simulink model "powerwindow_tl_v04"  (R2021a)
settings: Solver=ode1  StartTime=0.0  StopTime=20.0  FixedStep=0.01  RelTol=1e-3
PreLoadFcn:
  | if exist('tl_preloadfcn','file'), tl_preloadfcn(gcs,'22.1.0.27'); end
PostLoadFcn:
  | if exist('tl_postloadfcn','file'), tl_postloadfcn(gcs,'22.1.0.27'); end
InitFcn:
  | if exist('tlds_init','file'), tlds_init(gcs); end
StartFcn:
  | if exist('tlds_start','file'), tlds_start(gcs); end
StopFcn:
  | if exist('tlds_stop','file'), tlds_stop(gcs); end
undefined symbols (not defined in the file): auto_down_time, auto_up_time, emergency_down_time, position_endstop_top
libraries: tllib x7
(part 1 of 2)
PreSaveFcn:
  | if exist('tl_presavefcn','file'), tl_presavefcn(gcs); end
CloseFcn:
  | if exist('tl_closefcn','file'), tl_closefcn(gcs); end
settings Model: TL_MAIN_DATA={'codeopt',{'cleancode',1},'date',738946.6185320717,'advcodeopt',{'ExtendedBlockComments';'true'}}  DS_PROJECTFILE=powerwindow_tl_v01.dd  TLVersion=22.1.0.27  TL_GLOBAL_LOGGING_MODE=4  Creator=Wolfgang Meincke  LastModifiedBy=yatishc
settings SolverCC: AlgebraicLoopSolver=TrustRegion
settings DataIOCC: LimitDataPoints=on  SaveFormat=Array  ReturnWorkspaceOutputs=off
settings OptimizationCC: BlockReduction=off  BooleanDataType=off  ConditionallyExecuteInputs=off  OptimizeBlockIOStorage=off  BufferReuse=off  GlobalBufferReuse=off  ExpressionFolding=off  ExpressionDepthLimit=2147483647  LocalBlockOutputs=off  LifeSpan=inf  OptimizeDataStoreBuffers=off  BusAssignmentInplaceUpdate=off
settings DebuggingCC: SaveWithParameterizedLinksMsg=none  UnderspecifiedInitializationDetection=Classic  MergeDetectMultiDrivingBlocksExec=none  MultiTaskDSMMsg=warning  MultiTaskCondExecSysMsg=none  FcnCallInpInsideContextMsg=warning  UnconnectedInputMsg=none  UnconnectedOutputMsg=none  BusObjectLabelMismatch=error  StateNameClashWarn=warning  StrictBusMsg=ErrorOnBusTreatedAsVector  NonBusSignalsTreatedAsBus=error  SFUnexpectedBacktrackingDiag=warning  SFNoUnconditionalDefaultTransitionDiag=warning  SFMachineParentedDataDiag=warning  ArithmeticOperatorsInVariantConditions=warning
settings HardwareCC: ProdBitPerPointer=32  ProdBitPerSizeT=32  ProdBitPerPtrDiffT=32  ProdLargestAtomicFloat=None  ProdIntDivRoundTo=Undefined  ProdEndianess=Unspecified  ProdWordSize=32  ProdHWDeviceType=32-bit Generic
settings ModelReferenceCC: PropagateSignalLabelsOutOfModel=off
settings SFSimCC: SimUseLocalCustomCode=off  SimParseCustomCode=off  CustomCodeUndefinedFunction=UseInterfaceOnly
settings RTWCC: RTWUseLocalCustomCode=off
settings CodeAppCC: StateflowObjectComments=on
settings GRTTargetCC: TargetLangStandard=C89/C90 (ANSI)  CombineOutputUpdateFcns=off  GRTInterface=on
settings ConfigComp: CovMetricSettings=dw  CovSaveCumulativeToWorkspaceVar=on  CovSaveSingleToWorkspaceVar=on  CovExternalEMLEnable=off  CovSFcnEnable=off

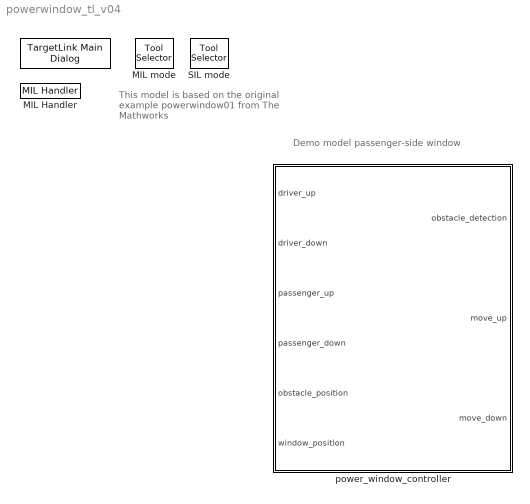
== system powerwindow_tl_v04 ==
  note: Demo model passenger-side window
  note: This model is based on the
      | original example powerwindow01
      | from The Mathworks
  " " : tllib/TargetLink Main Dialog  data=[]
      settings: SourceProductName=dSPACE TargetLink common blockset
  MIL Handler : tllib/MIL Handler  data={'date',730486}
      settings: SourceProductName=dSPACE TargetLink common blockset
  MIL mode : tllib/Tool Selector  Description=MIL\nmode  data={'date',730486}
      settings: SourceProductName=dSPACE TargetLink common blockset
  SIL mode : tllib/Tool Selector  Description=SIL\nmode  data={'date',730486}
      settings: SourceProductName=dSPACE TargetLink common blockset
  power_window_controller : Subsystem  Tag=TargetLink Simulation Frame  mask(TL_SimFrame){}
      settings: CopyFcn=if exist('tl_copyfcn','file'), tl_copyfcn(gcbh); end  NameChangeFcn=if exist('tl_framenamechangefcn','file'), tl_framenamechangefcn(gcbh); end
      settings: OpenFcn=|
      | if exist('open_tlsubsystem','file')
      |    open_tlsubsystem(gcbh);
      | else
      |    tlsubsystem = ...
      |       find_system(gcb, ...
      |       'LookUnderMasks','on', ...
      |       'FollowLinks','on', ...
      |       'Tag','MIL Subsystem');
      |    open_system(tlsubsystem);
      | end
      mask Display: disp('TargetLink\nModel-\nin-the-loop\nmode')

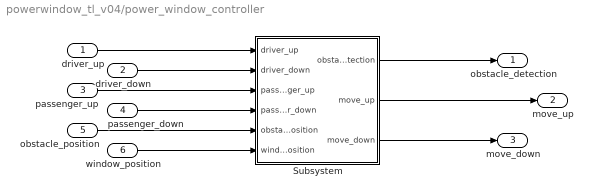
== system powerwindow_tl_v04/power_window_controller ==
  driver_up : Inport
  driver_down : Inport  Port=2
  passenger_up : Inport  Port=3
  passenger_down : Inport  Port=4
  obstacle_position : Inport  Port=5
  window_position : Inport  Port=6
  Subsystem : Subsystem  Tag=struct('sfcnName','power_window_controller_sf','subFunction','','srcSubsystem','')  mask(TL_Enable){}
      settings: OpenFcn=warndlg(get_param(gcb,'MaskHelp'),'Serious Warning');
      mask Help: This subsystem keeps the TargetLink subsystem (subsystem with TargetLink blocks for production code generation), and is needed for the TargetLink simulation frame to work properly. DO NOT DELETE OR MODIFY IT!
  obstacle_detection : Outport
  move_up : Outport  Port=2
  move_down : Outport  Port=3
  wires:
  driver_up/1 -> Subsystem/1(driver_up)
  driver_down/1 -> Subsystem/2(driver_down)
  passenger_up/1 -> Subsystem/3(passenger_up)
  passenger_down/1 -> Subsystem/4(passenger_down)
  obstacle_position/1 -> Subsystem/5(obstacle_position)
  window_position/1 -> Subsystem/6(window_position)
  Subsystem/1(obstacle_detection) -> obstacle_detection/1
  Subsystem/2(move_up) -> move_up/1
  Subsystem/3(move_down) -> move_down/1

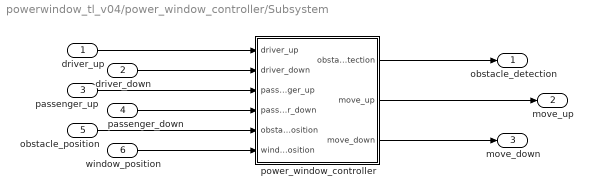
== system powerwindow_tl_v04/power_window_controller/Subsystem ==
  driver_up : Inport
  driver_down : Inport  Port=2
  passenger_up : Inport  Port=3
  passenger_down : Inport  Port=4
  obstacle_position : Inport  Port=5
  window_position : Inport  Port=6
  power_window_controller : Subsystem  Tag=MIL Subsystem  Description=a  RequirementInfo={} %GIDa_af814551_25fe_45fb_8d1f_eceee28b4185  LoadFcn=|
      | if exist('TargetLink.SimFrameHandler.TLSubsystem','class')
      |     TargetLink.SimFrameHandler.TLSubsystem.CreateWatchDog(gcbh);
      | end
      settings: CopyFcn=if exist('tl_copyfcn','file'), tl_copyfcn(gcbh); end  NameChangeFcn=if exist('tl_namechangefcn','file'), tl_namechangefcn(gcbh); end  DestroyFcn=if exist('update_tl_main_dlg','file'), update_tl_main_dlg('TL_subs_display'); end
      mask Display: disp('TargetLink Subsystem')
  obstacle_detection : Outport
  move_up : Outport  Port=2
  move_down : Outport  Port=3
  wires:
  driver_up/1 -> power_window_controller/1(driver_up)
  driver_down/1 -> power_window_controller/2(driver_down)
  passenger_up/1 -> power_window_controller/3(passenger_up)
  passenger_down/1 -> power_window_controller/4(passenger_down)
  obstacle_position/1 -> power_window_controller/5(obstacle_position)
  window_position/1 -> power_window_controller/6(window_position)
  power_window_controller/1(obstacle_detection) -> obstacle_detection/1
  power_window_controller/2(move_up) -> move_up/1
  power_window_controller/3(move_down) -> move_down/1

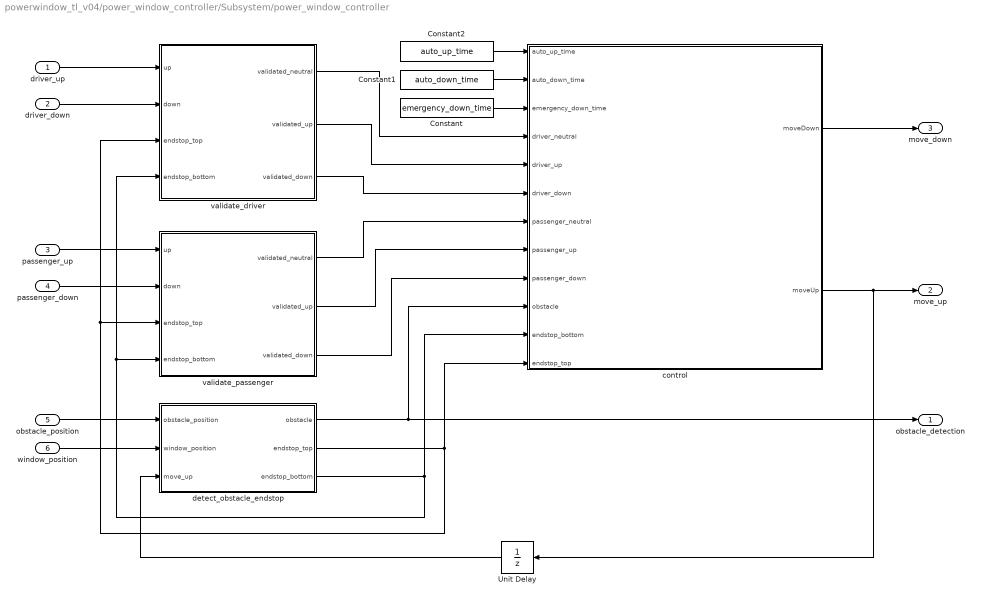
== system powerwindow_tl_v04/power_window_controller/Subsystem/power_window_controller ==
  driver_up : Inport  RequirementInfo={} %GIDa_659446e1_8e6d_43f9_b2fb_39d8267d7cb4  PortDimensions=1  mask(TL_Inport){data={'output',{'variable','Interface_Variables/driver_up'},'date',737859.75098331016}}
      settings: CopyFcn=if exist('copy_tlblock','file')==2,copy_tlblock(gcbh);end  DeleteFcn=if exist('delete_tlblock','file')==2,delete_tlblock(gcbh);end  NameChangeFcn=if exist('rename_tlblock','file')==2,rename_tlblock(gcbh);end  OpenFcn=if exist('tl_open_blockdlg','file')==2,tl_open_blockdlg(gcbh);else,open_system(gcbh,'parameter');end
      mask Help: eval(['if exist(''tl_online_help'',''file'') == 2, tl_online_help(''Topic'',''TL_Inport''),else, web([''jar:file:///'',matlabroot,''/help/toolbox/simulink/help.jar!/slref/' lower(get_param(gcbh,'Blocktype')) '.html''], ''-helpbrowser''),end'])
      mask Display:
      | [x,y] = tlDrawBrandOnBlockIcon(gcbh);
      | plot(x,y);
  driver_down : Inport  RequirementInfo={} %GIDa_1ab93b35_c370_40d7_8cfb_ac38c79443a8  Port=2  PortDimensions=1  mask(TL_Inport){data={'output',{'variable','Interface_Variables/driver_down'},'date',737859.75098344905}}
      settings: CopyFcn=if exist('copy_tlblock','file')==2,copy_tlblock(gcbh);end  DeleteFcn=if exist('delete_tlblock','file')==2,delete_tlblock(gcbh);end  NameChangeFcn=if exist('rename_tlblock','file')==2,rename_tlblock(gcbh);end  OpenFcn=if exist('tl_open_blockdlg','file')==2,tl_open_blockdlg(gcbh);else,open_system(gcbh,'parameter');end
      mask Help: eval(['if exist(''tl_online_help'',''file'') == 2, tl_online_help(''Topic'',''TL_Inport''),else, web([''jar:file:///'',matlabroot,''/help/toolbox/simulink/help.jar!/slref/' lower(get_param(gcbh,'Blocktype')) '.html''], ''-helpbrowser''),end'])
      mask Display:
      | [x,y] = tlDrawBrandOnBlockIcon(gcbh);
      | plot(x,y);
  passenger_up : Inport  RequirementInfo={} %GIDa_d69b69e4_dcf8_4d19_8e10_903162015345  Port=3  PortDimensions=1  mask(TL_Inport){data={'output',{'variable','Interface_Variables/passenger_up'},'date',737859.75098356477}}
      settings: CopyFcn=if exist('copy_tlblock','file')==2,copy_tlblock(gcbh);end  DeleteFcn=if exist('delete_tlblock','file')==2,delete_tlblock(gcbh);end  NameChangeFcn=if exist('rename_tlblock','file')==2,rename_tlblock(gcbh);end  OpenFcn=if exist('tl_open_blockdlg','file')==2,tl_open_blockdlg(gcbh);else,open_system(gcbh,'parameter');end
      mask Help: eval(['if exist(''tl_online_help'',''file'') == 2, tl_online_help(''Topic'',''TL_Inport''),else, web([''jar:file:///'',matlabroot,''/help/toolbox/simulink/help.jar!/slref/' lower(get_param(gcbh,'Blocktype')) '.html''], ''-helpbrowser''),end'])
      mask Display:
      | [x,y] = tlDrawBrandOnBlockIcon(gcbh);
      | plot(x,y);
  passenger_down : Inport  RequirementInfo={} %GIDa_ebdaa1c6_02ac_4284_94b9_7b936458029d  Port=4  PortDimensions=1  mask(TL_Inport){data={'output',{'variable','Interface_Variables/passenger_down'},'date',737859.7509836806}}
      settings: CopyFcn=if exist('copy_tlblock','file')==2,copy_tlblock(gcbh);end  DeleteFcn=if exist('delete_tlblock','file')==2,delete_tlblock(gcbh);end  NameChangeFcn=if exist('rename_tlblock','file')==2,rename_tlblock(gcbh);end  OpenFcn=if exist('tl_open_blockdlg','file')==2,tl_open_blockdlg(gcbh);else,open_system(gcbh,'parameter');end
      mask Help: eval(['if exist(''tl_online_help'',''file'') == 2, tl_online_help(''Topic'',''TL_Inport''),else, web([''jar:file:///'',matlabroot,''/help/toolbox/simulink/help.jar!/slref/' lower(get_param(gcbh,'Blocktype')) '.html''], ''-helpbrowser''),end'])
      mask Display:
      | [x,y] = tlDrawBrandOnBlockIcon(gcbh);
      | plot(x,y);
  obstacle_position : Inport  RequirementInfo={} %GIDa_3300e76c_dbcc_4aac_a719_94f0ce284986  Port=5  PortDimensions=1  mask(TL_Inport){data={'output',{'variable','Interface_Variables/obstacle_position'},'date',737859.75098381948}}
      settings: CopyFcn=if exist('copy_tlblock','file')==2,copy_tlblock(gcbh);end  DeleteFcn=if exist('delete_tlblock','file')==2,delete_tlblock(gcbh);end  NameChangeFcn=if exist('rename_tlblock','file')==2,rename_tlblock(gcbh);end  OpenFcn=if exist('tl_open_blockdlg','file')==2,tl_open_blockdlg(gcbh);else,open_system(gcbh,'parameter');end
      mask Help: eval(['if exist(''tl_online_help'',''file'') == 2, tl_online_help(''Topic'',''TL_Inport''),else, web([''jar:file:///'',matlabroot,''/help/toolbox/simulink/help.jar!/slref/' lower(get_param(gcbh,'Blocktype')) '.html''], ''-helpbrowser''),end'])
      mask Display:
      | [x,y] = tlDrawBrandOnBlockIcon(gcbh);
      | plot(x,y);
  window_position : Inport  RequirementInfo={} %GIDa_989a21e3_0ecd_4dda_a17a_2b6b96734fc1  Port=6  PortDimensions=1  mask(TL_Inport){data={'output',{'variable','Interface_Variables/window_position'},'autoscaling',{'mode',0},'date',738946.61852747691}}
      settings: CopyFcn=if exist('copy_tlblock','file')==2,copy_tlblock(gcbh);end  DeleteFcn=if exist('delete_tlblock','file')==2,delete_tlblock(gcbh);end  NameChangeFcn=if exist('rename_tlblock','file')==2,rename_tlblock(gcbh);end  OpenFcn=if exist('tl_open_blockdlg','file')==2,tl_open_blockdlg(gcbh);else,open_system(gcbh,'parameter');end
      mask Help: eval(['if exist(''tl_online_help'',''file'') == 2, tl_online_help(''Topic'',''TL_Inport''),else, web([''jar:file:///'',matlabroot,''/help/toolbox/simulink/help.jar!/slref/' lower(get_param(gcbh,'Blocktype')) '.html''], ''-helpbrowser''),end'])
      mask Display:
      | [x,y] = tlDrawBrandOnBlockIcon(gcbh);
      | plot(x,y);
  Constant : Constant  RequirementInfo={} %GIDa_956d11a9_9dab_432e_ba57_ca967d891d93  Value=emergency_down_time  mask(TL_Constant){data={'output',{'variable','Parameter/emergency_down_time'},'date',735993.41955673613}}
      settings: CopyFcn=if exist('copy_tlblock','file')==2,copy_tlblock(gcbh);end  DeleteFcn=if exist('delete_tlblock','file')==2,delete_tlblock(gcbh);end  NameChangeFcn=if exist('rename_tlblock','file')==2,rename_tlblock(gcbh);end  OpenFcn=if exist('tl_open_blockdlg','file')==2,tl_open_blockdlg(gcbh);else,open_system(gcbh,'parameter');end
      mask Help: eval(['if exist(''tl_online_help'',''file'') == 2, tl_online_help(''Topic'',''TL_Constant''),else, web([''jar:file:///'',matlabroot,''/help/toolbox/simulink/help.jar!/slref/' lower(get_param(gcbh,'Blocktype')) '.html''], ''-helpbrowser''),end'])
      mask Display:
      | [x,y] = tlDrawBrandOnBlockIcon(gcbh);
      | plot(x,y);
  Constant1 : Constant  RequirementInfo={} %GIDa_2751c770_b4bb_4dec_914d_687e5cb5d543  Value=auto_down_time  mask(TL_Constant){data={'output',{'variable','Parameter/auto_down_time'},'date',735993.41940997681}}
      settings: CopyFcn=if exist('copy_tlblock','file')==2,copy_tlblock(gcbh);end  DeleteFcn=if exist('delete_tlblock','file')==2,delete_tlblock(gcbh);end  NameChangeFcn=if exist('rename_tlblock','file')==2,rename_tlblock(gcbh);end  OpenFcn=if exist('tl_open_blockdlg','file')==2,tl_open_blockdlg(gcbh);else,open_system(gcbh,'parameter');end
      mask Help: eval(['if exist(''tl_online_help'',''file'') == 2, tl_online_help(''Topic'',''TL_Constant''),else, web([''jar:file:///'',matlabroot,''/help/toolbox/simulink/help.jar!/slref/' lower(get_param(gcbh,'Blocktype')) '.html''], ''-helpbrowser''),end'])
      mask Display:
      | [x,y] = tlDrawBrandOnBlockIcon(gcbh);
      | plot(x,y);
  Constant2 : Constant  RequirementInfo={} %GIDa_8b627733_7427_4dda_a61f_b41eab9425d8  Value=auto_up_time  mask(TL_Constant){data={'output',{'variable','Parameter/auto_up_time'},'date',735993.41923796292}}
      settings: CopyFcn=if exist('copy_tlblock','file')==2,copy_tlblock(gcbh);end  DeleteFcn=if exist('delete_tlblock','file')==2,delete_tlblock(gcbh);end  NameChangeFcn=if exist('rename_tlblock','file')==2,rename_tlblock(gcbh);end  OpenFcn=if exist('tl_open_blockdlg','file')==2,tl_open_blockdlg(gcbh);else,open_system(gcbh,'parameter');end
      mask Help: eval(['if exist(''tl_online_help'',''file'') == 2, tl_online_help(''Topic'',''TL_Constant''),else, web([''jar:file:///'',matlabroot,''/help/toolbox/simulink/help.jar!/slref/' lower(get_param(gcbh,'Blocktype')) '.html''], ''-helpbrowser''),end'])
      mask Display:
      | [x,y] = tlDrawBrandOnBlockIcon(gcbh);
      | plot(x,y);
  Unit Delay : UnitDelay  RequirementInfo={} %GIDa_93b85c05_e8a0_4dbe_a730_5e48319ef6b1  SampleTime=-1  HasFrameUpgradeWarning=on  mask(TL_UnitDelay){data={'output',{'inheritscaling',1},'date',735992.65481520828}}
      settings: CopyFcn=if exist('copy_tlblock','file')==2,copy_tlblock(gcbh);end  DeleteFcn=if exist('delete_tlblock','file')==2,delete_tlblock(gcbh);end  NameChangeFcn=if exist('rename_tlblock','file')==2,rename_tlblock(gcbh);end  OpenFcn=if exist('tl_open_blockdlg','file')==2,tl_open_blockdlg(gcbh);else,open_system(gcbh,'parameter');end
      mask Help: eval(['if exist(''tl_online_help'',''file'') == 2, tl_online_help(''Topic'',''TL_UnitDelay''),else, web([''jar:file:///'',matlabroot,''/help/toolbox/simulink/help.jar!/slref/' lower(get_param(gcbh,'Blocktype')) '.html''], ''-helpbrowser''),end'])
      mask Display:
      | [x,y] = tlDrawBrandOnBlockIcon(gcbh);
      | plot(x,y);
  control : Stateflow chart  RequirementInfo={} %GIDa_749aedb5_bc66_47f9_9eb4_81e35b8e797a  TreatAsAtomicUnit=on
  detect_obstacle_endstop : Subsystem  RequirementInfo={} %GIDa_31ce1ea2_9d98_4fb1_a59c_b951bb5150d4  TreatAsAtomicUnit=on
  validate_driver : Subsystem  RequirementInfo={} %GIDa_82511e6c_9958_497b_b695_db84d784c109  TreatAsAtomicUnit=on
  validate_passenger : Subsystem  RequirementInfo={} %GIDa_e14de864_d382_42e1_ae22_e1d99ae4970c  TreatAsAtomicUnit=on
  obstacle_detection : Outport  RequirementInfo={} %GIDa_ef03ae9f_d87c_4f06_8b3a_d815f18ae518  PortDimensions=1  mask(TL_Outport){data={'output',{'variable','Interface_Variables/obstacle_detection'},'date',737859.75098521996}}
      settings: CopyFcn=if exist('copy_tlblock','file')==2,copy_tlblock(gcbh);end  DeleteFcn=if exist('delete_tlblock','file')==2,delete_tlblock(gcbh);end  NameChangeFcn=if exist('rename_tlblock','file')==2,rename_tlblock(gcbh);end  OpenFcn=if exist('tl_open_blockdlg','file')==2,tl_open_blockdlg(gcbh);else,open_system(gcbh,'parameter');end
      mask Help: eval(['if exist(''tl_online_help'',''file'') == 2, tl_online_help(''Topic'',''TL_Outport''),else, web([''jar:file:///'',matlabroot,''/help/toolbox/simulink/help.jar!/slref/' lower(get_param(gcbh,'Blocktype')) '.html''], ''-helpbrowser''),end'])
      mask Display:
      | [x,y] = tlDrawBrandOnBlockIcon(gcbh);
      | plot(x,y);
  move_up : Outport  RequirementInfo={} %GIDa_416b2cf3_ac22_4bcc_a6db_f16da8ae98a0  Port=2  PortDimensions=1  mask(TL_Outport){data={'output',{'variable','Interface_Variables/move_up'},'date',738946.61852815968}}
      settings: CopyFcn=if exist('copy_tlblock','file')==2,copy_tlblock(gcbh);end  DeleteFcn=if exist('delete_tlblock','file')==2,delete_tlblock(gcbh);end  NameChangeFcn=if exist('rename_tlblock','file')==2,rename_tlblock(gcbh);end  OpenFcn=if exist('tl_open_blockdlg','file')==2,tl_open_blockdlg(gcbh);else,open_system(gcbh,'parameter');end
      mask Help: eval(['if exist(''tl_online_help'',''file'') == 2, tl_online_help(''Topic'',''TL_Outport''),else, web([''jar:file:///'',matlabroot,''/help/toolbox/simulink/help.jar!/slref/' lower(get_param(gcbh,'Blocktype')) '.html''], ''-helpbrowser''),end'])
      mask Display:
      | [x,y] = tlDrawBrandOnBlockIcon(gcbh);
      | plot(x,y);
  move_down : Outport  RequirementInfo={} %GIDa_bd818c14_0dbd_4464_a4c9_28139ad6e9fc  Port=3  PortDimensions=1  mask(TL_Outport){data={'output',{'variable','Interface_Variables/move_down'},'date',738946.6185283449}}
      settings: CopyFcn=if exist('copy_tlblock','file')==2,copy_tlblock(gcbh);end  DeleteFcn=if exist('delete_tlblock','file')==2,delete_tlblock(gcbh);end  NameChangeFcn=if exist('rename_tlblock','file')==2,rename_tlblock(gcbh);end  OpenFcn=if exist('tl_open_blockdlg','file')==2,tl_open_blockdlg(gcbh);else,open_system(gcbh,'parameter');end
      mask Help: eval(['if exist(''tl_online_help'',''file'') == 2, tl_online_help(''Topic'',''TL_Outport''),else, web([''jar:file:///'',matlabroot,''/help/toolbox/simulink/help.jar!/slref/' lower(get_param(gcbh,'Blocktype')) '.html''], ''-helpbrowser''),end'])
      mask Display:
      | [x,y] = tlDrawBrandOnBlockIcon(gcbh);
      | plot(x,y);
  wires:
  detect_obstacle_endstop/3(endstop_bottom) -> validate_passenger/4(endstop_bottom), validate_driver/4(endstop_bottom), control/11(endstop_bottom)
  detect_obstacle_endstop/2(endstop_top) -> validate_passenger/3(endstop_top), validate_driver/3(endstop_top), control/12(endstop_top)
  validate_passenger/3(validated_down) -> control/9(passenger_down)
  validate_passenger/2(validated_up) -> control/8(passenger_up)
  validate_passenger/1(validated_neutral) -> control/7(passenger_neutral)
  validate_driver/3(validated_down) -> control/6(driver_down)
  validate_driver/2(validated_up) -> control/5(driver_up)
  validate_driver/1(validated_neutral) -> control/4(driver_neutral)
  Constant/1 -> control/3(emergency_down_time)
  Constant1/1 -> control/2(auto_down_time)
  Constant2/1 -> control/1(auto_up_time)
  control/1(moveDown) -> move_down/1
  control/2(moveUp) -> Unit Delay/1, move_up/1
  detect_obstacle_endstop/1(obstacle) -> control/10(obstacle), obstacle_detection/1
  Unit Delay/1 -> detect_obstacle_endstop/3(move_up)
  window_position/1 -> detect_obstacle_endstop/2(window_position)
  obstacle_position/1 -> detect_obstacle_endstop/1(obstacle_position)
  passenger_down/1 -> validate_passenger/2(down)
  passenger_up/1 -> validate_passenger/1(up)
  driver_down/1 -> validate_driver/2(down)
  driver_up/1 -> validate_driver/1(up)

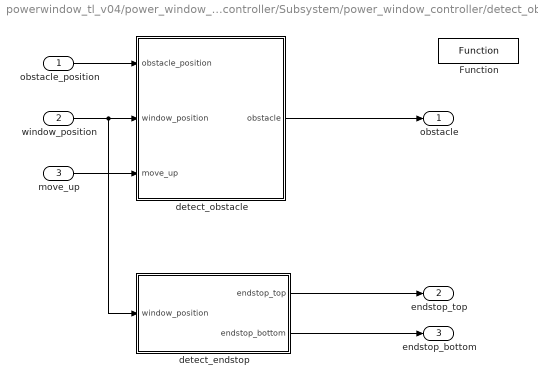
== system powerwindow_tl_v04/power_window_controller/Subsystem/power_window_controller/detect_obstacle_endstop ==
  obstacle_position : Inport  RequirementInfo={} %GIDa_8deb40d9_02a7_47d3_a077_a3d51c9036a6  mask(TL_Inport){data={'output',{'class','FCN_ARG','type','UInt16','scaling','position'},'autoscaling',{'mode',0},'date',737859.75098406256}}
      settings: CopyFcn=if exist('copy_tlblock','file')==2,copy_tlblock(gcbh);end  DeleteFcn=if exist('delete_tlblock','file')==2,delete_tlblock(gcbh);end  NameChangeFcn=if exist('rename_tlblock','file')==2,rename_tlblock(gcbh);end  OpenFcn=if exist('tl_open_blockdlg','file')==2,tl_open_blockdlg(gcbh);else,open_system(gcbh,'parameter');end
      mask Help: eval(['if exist(''tl_online_help'',''file'') == 2, tl_online_help(''Topic'',''TL_Inport''),else, web([''jar:file:///'',matlabroot,''/help/toolbox/simulink/help.jar!/slref/' lower(get_param(gcbh,'Blocktype')) '.html''], ''-helpbrowser''),end'])
      mask Display:
      | [x,y] = tlDrawBrandOnBlockIcon(gcbh);
      | plot(x,y);
  window_position : Inport  RequirementInfo={} %GIDa_3acd7b51_4611_4068_8b14_4157db533fe0  Port=2  mask(TL_Inport){data={'output',{'max',0.45,'min',0,'class','FCN_ARG','type','UInt16','scaling','position'},'autoscaling',{'mode',0},'date',737859.75098417827}}
      settings: CopyFcn=if exist('copy_tlblock','file')==2,copy_tlblock(gcbh);end  DeleteFcn=if exist('delete_tlblock','file')==2,delete_tlblock(gcbh);end  NameChangeFcn=if exist('rename_tlblock','file')==2,rename_tlblock(gcbh);end  OpenFcn=if exist('tl_open_blockdlg','file')==2,tl_open_blockdlg(gcbh);else,open_system(gcbh,'parameter');end
      mask Help: eval(['if exist(''tl_online_help'',''file'') == 2, tl_online_help(''Topic'',''TL_Inport''),else, web([''jar:file:///'',matlabroot,''/help/toolbox/simulink/help.jar!/slref/' lower(get_param(gcbh,'Blocktype')) '.html''], ''-helpbrowser''),end'])
      mask Display:
      | [x,y] = tlDrawBrandOnBlockIcon(gcbh);
      | plot(x,y);
  move_up : Inport  RequirementInfo={} %GIDa_dc6b20c7_b719_4404_84c6_3a7da964bb00  Port=3  mask(TL_Inport){data={'output',{'class','FCN_ARG','type','Bool'},'date',737859.75098429399}}
      settings: CopyFcn=if exist('copy_tlblock','file')==2,copy_tlblock(gcbh);end  DeleteFcn=if exist('delete_tlblock','file')==2,delete_tlblock(gcbh);end  NameChangeFcn=if exist('rename_tlblock','file')==2,rename_tlblock(gcbh);end  OpenFcn=if exist('tl_open_blockdlg','file')==2,tl_open_blockdlg(gcbh);else,open_system(gcbh,'parameter');end
      mask Help: eval(['if exist(''tl_online_help'',''file'') == 2, tl_online_help(''Topic'',''TL_Inport''),else, web([''jar:file:///'',matlabroot,''/help/toolbox/simulink/help.jar!/slref/' lower(get_param(gcbh,'Blocktype')) '.html''], ''-helpbrowser''),end'])
      mask Display:
      | [x,y] = tlDrawBrandOnBlockIcon(gcbh);
      | plot(x,y);
  Function : tllib/Function  RequirementInfo={} %GIDa_b7c77213_0814_4373_99ad_96eb40ab6c0b  data={'stepfunctionname','$B','codefile','$B','date',737859.75098562497}  displayString=FUNCTION
      settings: SourceProductName=dSPACE TargetLink common blockset
  detect_endstop : Subsystem  RequirementInfo={} %GIDa_d72c84c4_280a_4e28_b4ea_3d0c79734a93
  detect_obstacle : Subsystem  RequirementInfo={} %GIDa_bb01ba04_76a3_40a8_af03_45492fff9205
  obstacle : Outport  RequirementInfo={} %GIDa_1ed46e32_5fdf_43c3_b4c1_2e6fe11ea66d  mask(TL_Outport){data={'output',{'type','Bool'},'date',737859.75098456023}}
      settings: CopyFcn=if exist('copy_tlblock','file')==2,copy_tlblock(gcbh);end  DeleteFcn=if exist('delete_tlblock','file')==2,delete_tlblock(gcbh);end  NameChangeFcn=if exist('rename_tlblock','file')==2,rename_tlblock(gcbh);end  OpenFcn=if exist('tl_open_blockdlg','file')==2,tl_open_blockdlg(gcbh);else,open_system(gcbh,'parameter');end
      mask Help: eval(['if exist(''tl_online_help'',''file'') == 2, tl_online_help(''Topic'',''TL_Outport''),else, web([''jar:file:///'',matlabroot,''/help/toolbox/simulink/help.jar!/slref/' lower(get_param(gcbh,'Blocktype')) '.html''], ''-helpbrowser''),end'])
      mask Display:
      | [x,y] = tlDrawBrandOnBlockIcon(gcbh);
      | plot(x,y);
  endstop_top : Outport  RequirementInfo={} %GIDa_1a256a2f_5dd2_4087_bda5_0329f0d07827  Port=2  mask(TL_Outport){data={'output',{'type','Bool'},'date',737859.75098468747}}
      settings: CopyFcn=if exist('copy_tlblock','file')==2,copy_tlblock(gcbh);end  DeleteFcn=if exist('delete_tlblock','file')==2,delete_tlblock(gcbh);end  NameChangeFcn=if exist('rename_tlblock','file')==2,rename_tlblock(gcbh);end  OpenFcn=if exist('tl_open_blockdlg','file')==2,tl_open_blockdlg(gcbh);else,open_system(gcbh,'parameter');end
      mask Help: eval(['if exist(''tl_online_help'',''file'') == 2, tl_online_help(''Topic'',''TL_Outport''),else, web([''jar:file:///'',matlabroot,''/help/toolbox/simulink/help.jar!/slref/' lower(get_param(gcbh,'Blocktype')) '.html''], ''-helpbrowser''),end'])
      mask Display:
      | [x,y] = tlDrawBrandOnBlockIcon(gcbh);
      | plot(x,y);
  endstop_bottom : Outport  RequirementInfo={} %GIDa_6dec286d_6298_4408_b886_82a7527e3162  Port=3  mask(TL_Outport){data={'output',{'type','Bool'},'date',737859.75098481483}}
      settings: CopyFcn=if exist('copy_tlblock','file')==2,copy_tlblock(gcbh);end  DeleteFcn=if exist('delete_tlblock','file')==2,delete_tlblock(gcbh);end  NameChangeFcn=if exist('rename_tlblock','file')==2,rename_tlblock(gcbh);end  OpenFcn=if exist('tl_open_blockdlg','file')==2,tl_open_blockdlg(gcbh);else,open_system(gcbh,'parameter');end
      mask Help: eval(['if exist(''tl_online_help'',''file'') == 2, tl_online_help(''Topic'',''TL_Outport''),else, web([''jar:file:///'',matlabroot,''/help/toolbox/simulink/help.jar!/slref/' lower(get_param(gcbh,'Blocktype')) '.html''], ''-helpbrowser''),end'])
      mask Display:
      | [x,y] = tlDrawBrandOnBlockIcon(gcbh);
      | plot(x,y);
  wires:
  detect_endstop/2(endstop_bottom) -> endstop_bottom/1
  detect_endstop/1(endstop_top) -> endstop_top/1
  detect_obstacle/1(obstacle) -> obstacle/1
  obstacle_position/1 -> detect_obstacle/1(obstacle_position)
  window_position/1 -> detect_endstop/1(window_position), detect_obstacle/2(window_position)
  move_up/1 -> detect_obstacle/3(move_up)

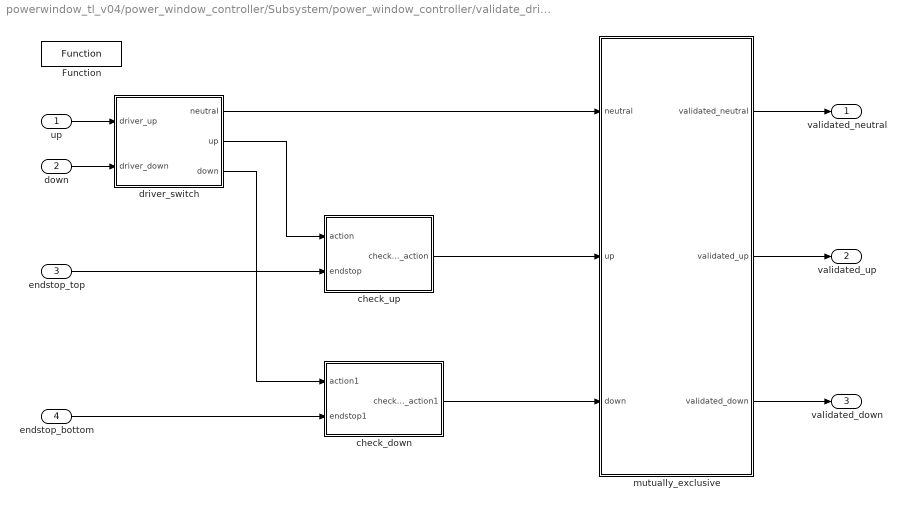
== system powerwindow_tl_v04/power_window_controller/Subsystem/power_window_controller/validate_driver ==
  up : Inport  RequirementInfo={} %GIDa_a086312e_84a9_4134_8fe8_58e6ae93af99
  down : Inport  RequirementInfo={} %GIDa_0d1ffd54_ad29_4e1f_882e_16153df02c8a  Port=2
  endstop_top : Inport  RequirementInfo={} %GIDa_781fb70f_52d8_4857_ba43_44cb3464c594  Port=3
  endstop_bottom : Inport  RequirementInfo={} %GIDa_e3b953a9_b457_4897_8b46_714a160c61cf  Port=4
  Function : tllib/Function  RequirementInfo={} %GIDa_54a5e059_d4de_4a84_9ac8_337f6a12dda9  data={'stepfunctionname','$B','codefile','$B','date',737859.75098574068}  displayString=FUNCTION
      settings: SourceProductName=dSPACE TargetLink common blockset
  check_down : Subsystem  RequirementInfo={} %GIDa_a4bdf102_4855_4528_91f0_1e0024cf733a
  check_up : Subsystem  RequirementInfo={} %GIDa_0c60c0e7_cf51_4c9a_91c0_2d7c796a2c30
  driver_switch : Subsystem  RequirementInfo={} %GIDa_209756ec_9b18_4a2d_9054_471e3f0ab27d
  mutually_exclusive : Subsystem  RequirementInfo={} %GIDa_1d3d9702_5b72_4bf0_b82b_e8ea1a7b6557
  validated_neutral : Outport  RequirementInfo={} %GIDa_c781003e_6df0_4b8a_b7a5_bffcf537bc74
  validated_up : Outport  RequirementInfo={} %GIDa_f238550d_e818_49a2_9c10_eb0ffa1ce5fb  Port=2
  validated_down : Outport  RequirementInfo={} %GIDa_dddc390a_ae46_45a4_bc1a_f28e24177265  Port=3
  wires:
  mutually_exclusive/3(validated_down) -> validated_down/1
  mutually_exclusive/2(validated_up) -> validated_up/1
  mutually_exclusive/1(validated_neutral) -> validated_neutral/1
  check_down/1(checked_action1) -> mutually_exclusive/3(down)
  check_up/1(checked_action) -> mutually_exclusive/2(up)
  driver_switch/1(neutral) -> mutually_exclusive/1(neutral)
  endstop_bottom/1 -> check_down/2(endstop1)
  endstop_top/1 -> check_up/2(endstop)
  driver_switch/3(down) -> check_down/1(action1)
  driver_switch/2(up) -> check_up/1(action)
  down/1 -> driver_switch/2(driver_down)
  up/1 -> driver_switch/1(driver_up)

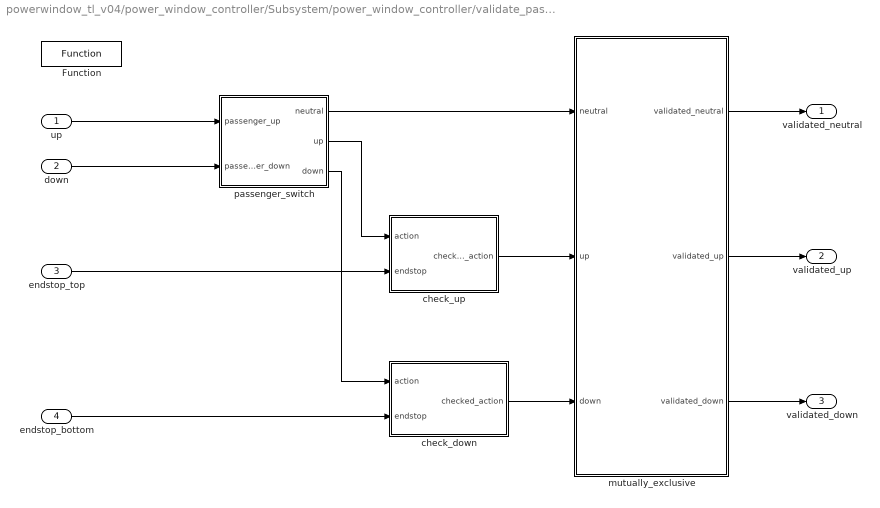
== system powerwindow_tl_v04/power_window_controller/Subsystem/power_window_controller/validate_passenger ==
  up : Inport  RequirementInfo={} %GIDa_f4ac5260_33b0_4aa8_b496_ce7dbde2b007
  down : Inport  RequirementInfo={} %GIDa_ca5488a3_7ad6_4747_b2c9_b68f9c5645f5  Port=2
  endstop_top : Inport  RequirementInfo={} %GIDa_21680e30_16f2_4234_a1ef_6a2080b73a81  Port=3
  endstop_bottom : Inport  RequirementInfo={} %GIDa_e852383a_3abb_449a_bd58_9f5bad2af98a  Port=4
  Function : tllib/Function  RequirementInfo={} %GIDa_df7a2d83_6608_49b8_9156_b1a02963e267  data={'stepfunctionname','$B','codefile','$B','date',737859.75098586804}  displayString=FUNCTION
      settings: SourceProductName=dSPACE TargetLink common blockset
  check_down : Subsystem  RequirementInfo={} %GIDa_a23ac263_65e6_424a_8985_470f15706266
  check_up : Subsystem  RequirementInfo={} %GIDa_8d89a62b_346d_4e97_a1a5_66ecfa3b145d
  mutually_exclusive : Subsystem  RequirementInfo={} %GIDa_9652364c_d107_41c5_b835_3aee88d1813d
  passenger_switch : Subsystem  RequirementInfo={} %GIDa_58f885c7_e073_4213_b989_f5990a4bd587
  validated_neutral : Outport  RequirementInfo={} %GIDa_71d2047f_12d8_48d3_8a1c_944a76cdb1a7
  validated_up : Outport  RequirementInfo={} %GIDa_becde808_ee45_42d7_b677_7eb470b8d02f  Port=2
  validated_down : Outport  RequirementInfo={} %GIDa_bc6a2113_7c48_4bb4_a262_3094ee2239cd  Port=3
  wires:
  mutually_exclusive/3(validated_down) -> validated_down/1
  mutually_exclusive/2(validated_up) -> validated_up/1
  mutually_exclusive/1(validated_neutral) -> validated_neutral/1
  check_down/1(checked_action) -> mutually_exclusive/3(down)
  check_up/1(checked_action) -> mutually_exclusive/2(up)
  passenger_switch/1(neutral) -> mutually_exclusive/1(neutral)
  endstop_bottom/1 -> check_down/2(endstop)
  endstop_top/1 -> check_up/2(endstop)
  passenger_switch/3(down) -> check_down/1(action)
  passenger_switch/2(up) -> check_up/1(action)
  down/1 -> passenger_switch/2(passenger_down)
  up/1 -> passenger_switch/1(passenger_up)

== system powerwindow_tl_v04/power_window_controller/Subsystem/power_window_controller/detect_obstacle_endstop/detect_endstop ==
  window_position : Inport  RequirementInfo={} %GIDa_894e360b_8fd2_4fc3_8fba_0f92be483dc0
  "Constant " : Constant  RequirementInfo={} %GIDa_0c389e23_b474_4c85_b75d_f78c722fba8b  Value=position_endstop_top  mask(TL_Constant){data={'output',{'variable','Parameter/position_endstop_top'},'date',735993.42899643513}}
      settings: CopyFcn=if exist('copy_tlblock','file')==2,copy_tlblock(gcbh);end  DeleteFcn=if exist('delete_tlblock','file')==2,delete_tlblock(gcbh);end  NameChangeFcn=if exist('rename_tlblock','file')==2,rename_tlblock(gcbh);end  OpenFcn=if exist('tl_open_blockdlg','file')==2,tl_open_blockdlg(gcbh);else,open_system(gcbh,'parameter');end
      mask Help: eval(['if exist(''tl_online_help'',''file'') == 2, tl_online_help(''Topic'',''TL_Constant''),else, web([''jar:file:///'',matlabroot,''/help/toolbox/simulink/help.jar!/slref/' lower(get_param(gcbh,'Blocktype')) '.html''], ''-helpbrowser''),end'])
      mask Display:
      | [x,y] = tlDrawBrandOnBlockIcon(gcbh);
      | plot(x,y);
  detection_endstop_bottom : RelationalOperator  RequirementInfo={} %GIDa_0cc291d9_85b6_47f8_bfbd_8cbe71d95b6d  Operator=<=  OutDataTypeStr=boolean  RndMeth=Nearest  mask(TL_RelationalOperator){data={'output',{'variable','Internal_Variables/detection_endstop_bottom'},'date',738946.61852846062}}
      settings: CopyFcn=if exist('copy_tlblock','file')==2,copy_tlblock(gcbh);end  DeleteFcn=if exist('delete_tlblock','file')==2,delete_tlblock(gcbh);end  NameChangeFcn=if exist('rename_tlblock','file')==2,rename_tlblock(gcbh);end  OpenFcn=if exist('tl_open_blockdlg','file')==2,tl_open_blockdlg(gcbh);else,open_system(gcbh,'parameter');end
      mask Help: eval(['if exist(''tl_online_help'',''file'') == 2, tl_online_help(''Topic'',''TL_RelationalOperator''),else, web([''jar:file:///'',matlabroot,''/help/toolbox/simulink/help.jar!/slref/' lower(get_param(gcbh,'Blocktype')) '.html''], ''-helpbrowser''),end'])
      mask Display:
      | [x,y] = tlDrawBrandOnBlockIcon(gcbh);
      | plot(x,y);
  detection_endstop_top : RelationalOperator  RequirementInfo={} %GIDa_e5434cca_dc39_45a0_84da_72791632bfd4  OutDataTypeStr=boolean  RndMeth=Nearest  mask(TL_RelationalOperator){data={'output',{'variable','Internal_Variables/detection_endstop_top'},'date',738946.61852854164}}
      settings: CopyFcn=if exist('copy_tlblock','file')==2,copy_tlblock(gcbh);end  DeleteFcn=if exist('delete_tlblock','file')==2,delete_tlblock(gcbh);end  NameChangeFcn=if exist('rename_tlblock','file')==2,rename_tlblock(gcbh);end  OpenFcn=if exist('tl_open_blockdlg','file')==2,tl_open_blockdlg(gcbh);else,open_system(gcbh,'parameter');end
      mask Help: eval(['if exist(''tl_online_help'',''file'') == 2, tl_online_help(''Topic'',''TL_RelationalOperator''),else, web([''jar:file:///'',matlabroot,''/help/toolbox/simulink/help.jar!/slref/' lower(get_param(gcbh,'Blocktype')) '.html''], ''-helpbrowser''),end'])
      mask Display:
      | [x,y] = tlDrawBrandOnBlockIcon(gcbh);
      | plot(x,y);
  position_endstop_bottom : Constant  RequirementInfo={} %GIDa_f99178ec_cdd7_40ba_af34_402563da826b  Value=0  mask(TL_Constant){data={'date',735992.66554090276}}
      settings: CopyFcn=if exist('copy_tlblock','file')==2,copy_tlblock(gcbh);end  DeleteFcn=if exist('delete_tlblock','file')==2,delete_tlblock(gcbh);end  NameChangeFcn=if exist('rename_tlblock','file')==2,rename_tlblock(gcbh);end  OpenFcn=if exist('tl_open_blockdlg','file')==2,tl_open_blockdlg(gcbh);else,open_system(gcbh,'parameter');end
      mask Help: eval(['if exist(''tl_online_help'',''file'') == 2, tl_online_help(''Topic'',''TL_Constant''),else, web([''jar:file:///'',matlabroot,''/help/toolbox/simulink/help.jar!/slref/' lower(get_param(gcbh,'Blocktype')) '.html''], ''-helpbrowser''),end'])
      mask Display:
      | [x,y] = tlDrawBrandOnBlockIcon(gcbh);
      | plot(x,y);
  endstop_top : Outport  RequirementInfo={} %GIDa_ffb08f70_d85d_4850_be6f_7bb91d3cfdde
  endstop_bottom : Outport  RequirementInfo={} %GIDa_8d02e7ce_a78c_4d52_b3b2_002530073764  Port=2
  wires:
  detection_endstop_bottom/1 -> endstop_bottom/1  "endstop_bottom"
  detection_endstop_top/1 -> endstop_top/1  "endstop_top"
  position_endstop_bottom/1 -> detection_endstop_bottom/2
  window_position/1 -> detection_endstop_bottom/1, detection_endstop_top/1
  "Constant "/1 -> detection_endstop_top/2

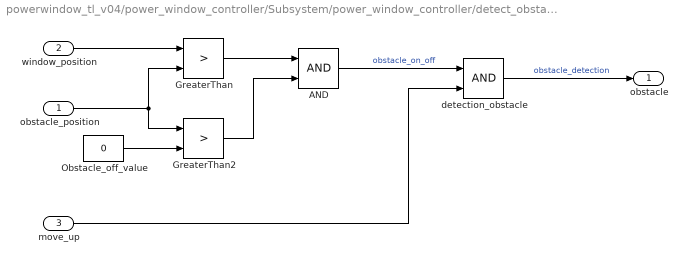
== system powerwindow_tl_v04/power_window_controller/Subsystem/power_window_controller/detect_obstacle_endstop/detect_obstacle ==
  obstacle_position : Inport  RequirementInfo={} %GIDa_d8b8744d_8ba1_4043_9716_81593ba4d7ee
  window_position : Inport  RequirementInfo={} %GIDa_84d6c3d8_9214_4b6f_bb44_466e022ad5b9  Port=2
  move_up : Inport  RequirementInfo={} %GIDa_af70ce51_e34d_4539_828d_91355b704b56  Port=3
  AND : Logic  RequirementInfo={} %GIDa_43bca29f_752d_4258_8419_864b7cd459a5  AllPortsSameDT=off  OutDataTypeStr=boolean  mask(TL_LogicalOperator){data={'date',730486}}
      settings: CopyFcn=if exist('copy_tlblock','file')==2,copy_tlblock(gcbh);end  DeleteFcn=if exist('delete_tlblock','file')==2,delete_tlblock(gcbh);end  NameChangeFcn=if exist('rename_tlblock','file')==2,rename_tlblock(gcbh);end  OpenFcn=if exist('tl_open_blockdlg','file')==2,tl_open_blockdlg(gcbh);else,open_system(gcbh,'parameter');end
      mask Help: eval(['if exist(''tl_online_help'',''file'') == 2, tl_online_help(''Topic'',''TL_LogicalOperator''),else, web([''jar:file:///'',matlabroot,''/help/toolbox/simulink/help.jar!/slref/' lower(get_param(gcbh,'Blocktype')) '.html''], ''-helpbrowser''),end'])
      mask Display:
      | [x,y] = tlDrawBrandOnBlockIcon(gcbh);
      | plot(x,y);
  "GreaterThan  " : RelationalOperator  RequirementInfo={} %GIDa_3f5b6ad9_5781_40f9_99a2_c74226edfde4  Operator=>  OutDataTypeStr=boolean  RndMeth=Nearest  mask(TL_RelationalOperator){data={'date',735992.6592954282}}
      settings: CopyFcn=if exist('copy_tlblock','file')==2,copy_tlblock(gcbh);end  DeleteFcn=if exist('delete_tlblock','file')==2,delete_tlblock(gcbh);end  NameChangeFcn=if exist('rename_tlblock','file')==2,rename_tlblock(gcbh);end  OpenFcn=if exist('tl_open_blockdlg','file')==2,tl_open_blockdlg(gcbh);else,open_system(gcbh,'parameter');end
      mask Help: eval(['if exist(''tl_online_help'',''file'') == 2, tl_online_help(''Topic'',''TL_RelationalOperator''),else, web([''jar:file:///'',matlabroot,''/help/toolbox/simulink/help.jar!/slref/' lower(get_param(gcbh,'Blocktype')) '.html''], ''-helpbrowser''),end'])
      mask Display:
      | [x,y] = tlDrawBrandOnBlockIcon(gcbh);
      | plot(x,y);
  GreaterThan2 : RelationalOperator  RequirementInfo={} %GIDa_714d93c7_31c7_4861_8788_47d721e53c9c  Operator=>  OutDataTypeStr=boolean  RndMeth=Nearest  mask(TL_RelationalOperator){data={'date',735992.65940515045}}
      settings: CopyFcn=if exist('copy_tlblock','file')==2,copy_tlblock(gcbh);end  DeleteFcn=if exist('delete_tlblock','file')==2,delete_tlblock(gcbh);end  NameChangeFcn=if exist('rename_tlblock','file')==2,rename_tlblock(gcbh);end  OpenFcn=if exist('tl_open_blockdlg','file')==2,tl_open_blockdlg(gcbh);else,open_system(gcbh,'parameter');end
      mask Help: eval(['if exist(''tl_online_help'',''file'') == 2, tl_online_help(''Topic'',''TL_RelationalOperator''),else, web([''jar:file:///'',matlabroot,''/help/toolbox/simulink/help.jar!/slref/' lower(get_param(gcbh,'Blocktype')) '.html''], ''-helpbrowser''),end'])
      mask Display:
      | [x,y] = tlDrawBrandOnBlockIcon(gcbh);
      | plot(x,y);
  Obstacle_off_value : Constant  RequirementInfo={} %GIDa_b7ef5796_dc21_4330_9187_1ce64823c5ee  Value=0  mask(TL_Constant){data={'date',735992.66084980324}}
      settings: CopyFcn=if exist('copy_tlblock','file')==2,copy_tlblock(gcbh);end  DeleteFcn=if exist('delete_tlblock','file')==2,delete_tlblock(gcbh);end  NameChangeFcn=if exist('rename_tlblock','file')==2,rename_tlblock(gcbh);end  OpenFcn=if exist('tl_open_blockdlg','file')==2,tl_open_blockdlg(gcbh);else,open_system(gcbh,'parameter');end
      mask Help: eval(['if exist(''tl_online_help'',''file'') == 2, tl_online_help(''Topic'',''TL_Constant''),else, web([''jar:file:///'',matlabroot,''/help/toolbox/simulink/help.jar!/slref/' lower(get_param(gcbh,'Blocktype')) '.html''], ''-helpbrowser''),end'])
      mask Display:
      | [x,y] = tlDrawBrandOnBlockIcon(gcbh);
      | plot(x,y);
  detection_obstacle : Logic  RequirementInfo={} %GIDa_2e6d66e5_5050_44b5_ab2e_fbf53bc38c2b  AllPortsSameDT=off  OutDataTypeStr=boolean  mask(TL_LogicalOperator){data={'output',{'variable','Internal_Variables/detection_obstacle'},'date',738946.61852778937}}
      settings: CopyFcn=if exist('copy_tlblock','file')==2,copy_tlblock(gcbh);end  DeleteFcn=if exist('delete_tlblock','file')==2,delete_tlblock(gcbh);end  NameChangeFcn=if exist('rename_tlblock','file')==2,rename_tlblock(gcbh);end  OpenFcn=if exist('tl_open_blockdlg','file')==2,tl_open_blockdlg(gcbh);else,open_system(gcbh,'parameter');end
      mask Help: eval(['if exist(''tl_online_help'',''file'') == 2, tl_online_help(''Topic'',''TL_LogicalOperator''),else, web([''jar:file:///'',matlabroot,''/help/toolbox/simulink/help.jar!/slref/' lower(get_param(gcbh,'Blocktype')) '.html''], ''-helpbrowser''),end'])
      mask Display:
      | [x,y] = tlDrawBrandOnBlockIcon(gcbh);
      | plot(x,y);
  obstacle : Outport  RequirementInfo={} %GIDa_79cffe66_5440_4d26_b2b6_3b52a3647c61
  wires:
  Obstacle_off_value/1 -> GreaterThan2/2
  obstacle_position/1 -> "GreaterThan  "/2, GreaterThan2/1
  GreaterThan2/1 -> AND/2
  move_up/1 -> detection_obstacle/2
  AND/1 -> detection_obstacle/1  "obstacle_on_off"
  "GreaterThan  "/1 -> AND/1
  window_position/1 -> "GreaterThan  "/1
  detection_obstacle/1 -> obstacle/1  "obstacle_detection"

== system powerwindow_tl_v04/power_window_controller/Subsystem/power_window_controller/validate_driver/check_down ==
  action1 : Inport  RequirementInfo={} %GIDa_ea5cc4fd_4531_4818_94f6_19cbb6feae29
  endstop1 : Inport  RequirementInfo={} %GIDa_78fae135_5c28_493a_839f_69269fbea1c2  Port=2
  Logical Operator : Logic  AllPortsSameDT=off  OutDataTypeStr=boolean  mask(TL_LogicalOperator){data={'date',735997.67236332176}}
      settings: CopyFcn=if exist('copy_tlblock','file')==2,copy_tlblock(gcbh);end  DeleteFcn=if exist('delete_tlblock','file')==2,delete_tlblock(gcbh);end  NameChangeFcn=if exist('rename_tlblock','file')==2,rename_tlblock(gcbh);end  OpenFcn=if exist('tl_open_blockdlg','file')==2,tl_open_blockdlg(gcbh);else,open_system(gcbh,'parameter');end
      mask Help: eval(['if exist(''tl_online_help'',''file'') == 2, tl_online_help(''Topic'',''TL_LogicalOperator''),else, web([''jar:file:///'',matlabroot,''/help/toolbox/simulink/help.jar!/slref/' lower(get_param(gcbh,'Blocktype')) '.html''], ''-helpbrowser''),end'])
      mask Display:
      | [x,y] = tlDrawBrandOnBlockIcon(gcbh);
      | plot(x,y);
  Logical Operator1 : Logic  Operator=NOT  Inputs=1  AllPortsSameDT=off  OutDataTypeStr=boolean  mask(TL_LogicalOperator){data={'date',735997.67261783569}}
      settings: CopyFcn=if exist('copy_tlblock','file')==2,copy_tlblock(gcbh);end  DeleteFcn=if exist('delete_tlblock','file')==2,delete_tlblock(gcbh);end  NameChangeFcn=if exist('rename_tlblock','file')==2,rename_tlblock(gcbh);end  OpenFcn=if exist('tl_open_blockdlg','file')==2,tl_open_blockdlg(gcbh);else,open_system(gcbh,'parameter');end
      mask Help: eval(['if exist(''tl_online_help'',''file'') == 2, tl_online_help(''Topic'',''TL_LogicalOperator''),else, web([''jar:file:///'',matlabroot,''/help/toolbox/simulink/help.jar!/slref/' lower(get_param(gcbh,'Blocktype')) '.html''], ''-helpbrowser''),end'])
      mask Display:
      | [x,y] = tlDrawBrandOnBlockIcon(gcbh);
      | plot(x,y);
  checked_action1 : Outport  RequirementInfo={} %GIDa_e5d57404_6a5d_416a_a3cc_34eb56a63336
  wires:
  action1/1 -> Logical Operator/1
  Logical Operator1/1 -> Logical Operator/2
  Logical Operator/1 -> checked_action1/1
  endstop1/1 -> Logical Operator1/1

== system powerwindow_tl_v04/power_window_controller/Subsystem/power_window_controller/validate_driver/check_up ==
  action : Inport  RequirementInfo={} %GIDa_a5dd46b4_51cd_4488_99aa_012cdf4e3921
  endstop : Inport  RequirementInfo={} %GIDa_8a8450a4_4afa_487b_b3ab_f7ceeaf7bd02  Port=2
  allow_action : Logic  RequirementInfo={} %GIDa_d5fb3aa3_08b9_4f34_a35e_58c022df2a44  AllPortsSameDT=off  OutDataTypeStr=boolean  mask(TL_LogicalOperator){data={'date',730486}}
      settings: CopyFcn=if exist('copy_tlblock','file')==2,copy_tlblock(gcbh);end  DeleteFcn=if exist('delete_tlblock','file')==2,delete_tlblock(gcbh);end  NameChangeFcn=if exist('rename_tlblock','file')==2,rename_tlblock(gcbh);end  OpenFcn=if exist('tl_open_blockdlg','file')==2,tl_open_blockdlg(gcbh);else,open_system(gcbh,'parameter');end
      mask Help: eval(['if exist(''tl_online_help'',''file'') == 2, tl_online_help(''Topic'',''TL_LogicalOperator''),else, web([''jar:file:///'',matlabroot,''/help/toolbox/simulink/help.jar!/slref/' lower(get_param(gcbh,'Blocktype')) '.html''], ''-helpbrowser''),end'])
      mask Display:
      | [x,y] = tlDrawBrandOnBlockIcon(gcbh);
      | plot(x,y);
  not : Logic  RequirementInfo={} %GIDa_d2bbe0cd_d82d_411b_ad5e_b27c208d24b8  Operator=NOT  Inputs=1  AllPortsSameDT=off  OutDataTypeStr=boolean  mask(TL_LogicalOperator){data={'date',735992.62481011578}}
      settings: CopyFcn=if exist('copy_tlblock','file')==2,copy_tlblock(gcbh);end  DeleteFcn=if exist('delete_tlblock','file')==2,delete_tlblock(gcbh);end  NameChangeFcn=if exist('rename_tlblock','file')==2,rename_tlblock(gcbh);end  OpenFcn=if exist('tl_open_blockdlg','file')==2,tl_open_blockdlg(gcbh);else,open_system(gcbh,'parameter');end
      mask Help: eval(['if exist(''tl_online_help'',''file'') == 2, tl_online_help(''Topic'',''TL_LogicalOperator''),else, web([''jar:file:///'',matlabroot,''/help/toolbox/simulink/help.jar!/slref/' lower(get_param(gcbh,'Blocktype')) '.html''], ''-helpbrowser''),end'])
      mask Display:
      | [x,y] = tlDrawBrandOnBlockIcon(gcbh);
      | plot(x,y);
  checked_action : Outport  RequirementInfo={} %GIDa_4de0fac3_8aaa_4223_a9d2_8c3216f59239
  wires:
  not/1 -> allow_action/2
  endstop/1 -> not/1
  action/1 -> allow_action/1
  allow_action/1 -> checked_action/1  "checked_action"

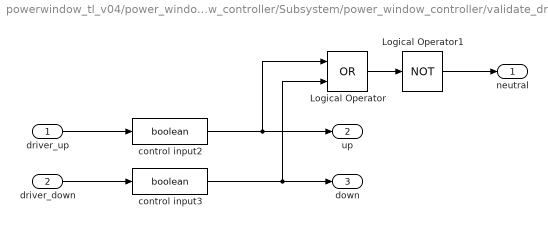
== system powerwindow_tl_v04/power_window_controller/Subsystem/power_window_controller/validate_driver/driver_switch ==
  driver_up : Inport  RequirementInfo={} %GIDa_457d0bab_1a2f_4276_adb6_bd1f39708df7
  driver_down : Inport  RequirementInfo={} %GIDa_529db648_4fe5_4c58_98e1_11397fc73a63  Port=2
  Logical Operator : Logic  RequirementInfo={} %GIDa_41bc118a_bf95_4afc_8d02_fd18bbf041ef  Operator=OR  AllPortsSameDT=off  OutDataTypeStr=boolean  mask(TL_LogicalOperator){data={'date',735992.62219250004}}
      settings: CopyFcn=if exist('copy_tlblock','file')==2,copy_tlblock(gcbh);end  DeleteFcn=if exist('delete_tlblock','file')==2,delete_tlblock(gcbh);end  NameChangeFcn=if exist('rename_tlblock','file')==2,rename_tlblock(gcbh);end  OpenFcn=if exist('tl_open_blockdlg','file')==2,tl_open_blockdlg(gcbh);else,open_system(gcbh,'parameter');end
      mask Help: eval(['if exist(''tl_online_help'',''file'') == 2, tl_online_help(''Topic'',''TL_LogicalOperator''),else, web([''jar:file:///'',matlabroot,''/help/toolbox/simulink/help.jar!/slref/' lower(get_param(gcbh,'Blocktype')) '.html''], ''-helpbrowser''),end'])
      mask Display:
      | [x,y] = tlDrawBrandOnBlockIcon(gcbh);
      | plot(x,y);
  Logical Operator1 : Logic  RequirementInfo={} %GIDa_ba497dfd_e5b5_4976_9463_f13d3dacf120  Operator=NOT  Inputs=1  AllPortsSameDT=off  OutDataTypeStr=boolean  mask(TL_LogicalOperator){data={'date',735992.62266063655}}
      settings: CopyFcn=if exist('copy_tlblock','file')==2,copy_tlblock(gcbh);end  DeleteFcn=if exist('delete_tlblock','file')==2,delete_tlblock(gcbh);end  NameChangeFcn=if exist('rename_tlblock','file')==2,rename_tlblock(gcbh);end  OpenFcn=if exist('tl_open_blockdlg','file')==2,tl_open_blockdlg(gcbh);else,open_system(gcbh,'parameter');end
      mask Help: eval(['if exist(''tl_online_help'',''file'') == 2, tl_online_help(''Topic'',''TL_LogicalOperator''),else, web([''jar:file:///'',matlabroot,''/help/toolbox/simulink/help.jar!/slref/' lower(get_param(gcbh,'Blocktype')) '.html''], ''-helpbrowser''),end'])
      mask Display:
      | [x,y] = tlDrawBrandOnBlockIcon(gcbh);
      | plot(x,y);
  control input2 : DataTypeConversion  RequirementInfo={} %GIDa_97663cca_2510_4ce5_9bd9_432eef1ac42a  OutDataTypeStr=boolean  SaturateOnIntegerOverflow=on  RndMeth=Zero  mask(TL_Rescaler){data={'date',730486}}
      settings: CopyFcn=if exist('copy_tlblock','file')==2,copy_tlblock(gcbh);end  DeleteFcn=if exist('delete_tlblock','file')==2,delete_tlblock(gcbh);end  NameChangeFcn=if exist('rename_tlblock','file')==2,rename_tlblock(gcbh);end  OpenFcn=if exist('tl_open_blockdlg','file')==2,tl_open_blockdlg(gcbh);else,open_system(gcbh,'parameter');end
      mask Help: eval(['if exist(''tl_online_help'',''file'') == 2, tl_online_help(''Topic'',''TL_Rescaler''),else, web([''jar:file:///'',matlabroot,''/help/toolbox/simulink/help.jar!/slref/' lower(get_param(gcbh,'Blocktype')) '.html''], ''-helpbrowser''),end'])
      mask Display:
      | [x,y] = tlDrawBrandOnBlockIcon(gcbh);
      | plot(x,y);
  control input3 : DataTypeConversion  RequirementInfo={} %GIDa_ea81ae5a_fed2_4093_befb_3b4eb6247037  OutDataTypeStr=boolean  SaturateOnIntegerOverflow=on  RndMeth=Zero  mask(TL_Rescaler){data={'date',730486}}
      settings: CopyFcn=if exist('copy_tlblock','file')==2,copy_tlblock(gcbh);end  DeleteFcn=if exist('delete_tlblock','file')==2,delete_tlblock(gcbh);end  NameChangeFcn=if exist('rename_tlblock','file')==2,rename_tlblock(gcbh);end  OpenFcn=if exist('tl_open_blockdlg','file')==2,tl_open_blockdlg(gcbh);else,open_system(gcbh,'parameter');end
      mask Help: eval(['if exist(''tl_online_help'',''file'') == 2, tl_online_help(''Topic'',''TL_Rescaler''),else, web([''jar:file:///'',matlabroot,''/help/toolbox/simulink/help.jar!/slref/' lower(get_param(gcbh,'Blocktype')) '.html''], ''-helpbrowser''),end'])
      mask Display:
      | [x,y] = tlDrawBrandOnBlockIcon(gcbh);
      | plot(x,y);
  neutral : Outport  RequirementInfo={} %GIDa_8a843187_86a2_4816_ba63_473f86f3416f
  up : Outport  RequirementInfo={} %GIDa_838b3e71_ca14_41ba_a061_b40b0627434f  Port=2
  down : Outport  RequirementInfo={} %GIDa_3f496670_696b_49bd_98bc_9983f12010cf  Port=3
  wires:
  Logical Operator1/1 -> neutral/1
  Logical Operator/1 -> Logical Operator1/1
  control input3/1 -> Logical Operator/2, down/1
  control input2/1 -> Logical Operator/1, up/1
  driver_down/1 -> control input3/1
  driver_up/1 -> control input2/1
